simulink model "FullFilterTest_testJ"  (R2020a)
settings: Solver=ode3  StartTime=0.0  StopTime=100  FixedStep=1  RelTol=1e-3
libraries: aerolibconvert2 x1, simulink x1, sharedutil x1, sharedtransform x1
settings Model: Creator=pieterpinson  LastModifiedBy=jamie
settings DataIOCC: SaveFormat=StructureWithTime
settings OptimizationCC: LifeSpan=inf
settings DebuggingCC: SFExecutionAtInitializationDiag=none  ArithmeticOperatorsInVariantConditions=warning
settings HardwareCC: ProdBitPerSizeT=32  ProdBitPerPtrDiffT=32  ProdWordSize=32  ProdHWDeviceType=Specified
settings SFSimCC: CustomCodeUndefinedFunction=UseInterfaceOnly
settings CodeAppCC: StateflowObjectComments=on

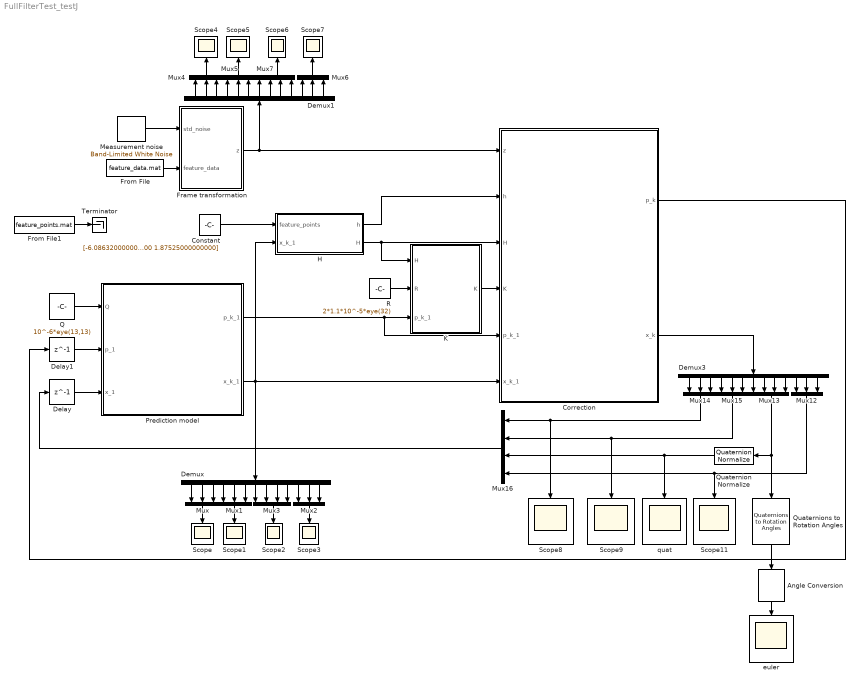
== system FullFilterTest_testJ ==
  Angle Conversion : aerolibconvert2/Angle Conversion  IU=rad  OU=deg
  Constant : Constant  Value=|
      | [-6.08632000000000	-6.29117000000000	-6.23068000000000	-6.17018000000000	0.665410000000000	0.665410000000000	2.50061000000000	2.48017000000000	6.23068000000000	6.35166000000000	6.35166000000000	6.29117000000000	10.8457800000000	10.8280700000000	29.5266400000000	29.5582500000000;
      | -0.635730000000000	1.88967000000000	-0.602200000000000	1.85389000000000	2.17147000000000	2.18343000000000	3.10581000000000	3.09464000000000	-0.636800000000000	2.53604000000000	-0.625630000000000	2.54752000000000	2.60307000000000	1.32946000000000	-8.00742000000000	-9.30518000000000;
      | -1.81476000000000	-1.81476000000000	1.87525000000000	1.93574000000000	7.31953000000000	-7.38003000000000	-7.25904000000000	7.31953000000000	1.93574000000000	2.05673000000000	-1.81476000000000	-1.93574000000000	-3.56903000000000	3.69001000000000	-5.38379000000000	1.87525000000000]
  Correction : MATLAB Function  TreatAsAtomicUnit=on
  Delay : Delay  DelayLength=1  InitialCondition=|
      | [-0.0019 ; 0.0017 ; 1.0891 ; 0 ; 0 ; 0 ; -0.7226 ; 0.6358 ; 0.1434 ; 0.2302
      | ; -0.0873 ; -0.1489 ; 0.0262]
  Delay1 : Delay  DelayLength=1  InitialCondition=100*10*diag([1,1,2,0.01,0.01,0.01,0.01,0.01,0.01,0.01,0.01,0.01,0.01])
  Demux : Demux  Outputs=13
  Demux1 : Demux  Outputs=13
  Demux3 : Demux  Outputs=13
  Frame transformation : MATLAB Function  TreatAsAtomicUnit=on
  From File : FromFile  FileName=feature_data.mat  SampleTime=1
  From File1 : FromFile  FileName=feature_points.mat  SampleTime=0
  H : MATLAB Function  TreatAsAtomicUnit=on
  K : MATLAB Function  TreatAsAtomicUnit=on
  Measurement noise : simulink/Sources/Band-Limited White Noise  Cov=[sin(sin(0.1))]  Ts=1  seed=[23341]
  Mux{,1..2,4..6,12,14..15} (9 alike) : Mux  Inputs=3
  Mux{3,7,13,16} (4 alike) : Mux
  Prediction model : MATLAB Function  TreatAsAtomicUnit=on
  Q : Constant  Value=10^-6*eye(13,13)
  Quaternion Normalize : sharedutil/Quaternion Normalize  aMode=aMode
      settings: SourceProductBaseCode=AE,PW,MT,VE,VP
  Quaternions to Rotation Angles : sharedtransform/Quaternions to Rotation Angles  rotationOrder=ZYX  aMode=aMode
      settings: SourceProductBaseCode=AE,PW,MT,VE,VP
  R : Constant  Value=2*1.1*10^-5*eye(32)
  Scope{,1..9,11} (11 alike) : Scope
  Terminator : Terminator
  euler : Scope
  quat : Scope
  wires:
  Prediction model/2(x_k_1) -> H/2(x_k_1), Correction/6(x_k_1), Demux/1
  Mux3/1 -> Scope2/1
  Demux/13 -> Mux2/3
  Demux/12 -> Mux2/2
  Demux/11 -> Mux2/1
  Demux/10 -> Mux3/4
  Demux/9 -> Mux3/3
  Demux/8 -> Mux3/2
  Demux/7 -> Mux3/1
  Demux/6 -> Mux1/3
  Demux/5 -> Mux1/2
  Demux/4 -> Mux1/1
  Demux/3 -> Mux/3
  Demux/2 -> Mux/2
  Demux/1 -> Mux/1
  Mux1/1 -> Scope1/1
  Mux/1 -> Scope/1
  Delay/1 -> Prediction model/3(x_1)
  Mux2/1 -> Scope3/1
  Q/1 -> Prediction model/1(Q)
  Delay1/1 -> Prediction model/2(p_1)
  Mux6/1 -> Scope7/1
  Demux1/3 -> Mux4/3
  Demux1/10 -> Mux7/4
  Demux1/2 -> Mux4/2
  Demux1/1 -> Mux4/1
  Demux1/11 -> Mux6/1
  Mux4/1 -> Scope4/1
  Mux5/1 -> Scope5/1
  Mux7/1 -> Scope6/1
  Demux1/6 -> Mux5/3
  Demux1/9 -> Mux7/3
  Demux1/13 -> Mux6/3
  Demux1/12 -> Mux6/2
  Demux1/7 -> Mux7/1
  Frame transformation/1(z) -> Correction/1(z), Demux1/1
  Demux1/4 -> Mux5/1
  Demux1/5 -> Mux5/2
  Demux1/8 -> Mux7/2
  H/2(H) -> Correction/3(H), K/1(H)
  Correction/1(p_k) -> Delay1/1
  Correction/2(x_k) -> Demux3/1
  Prediction model/1(p_k_1) -> Correction/5(p_k_1), K/3(p_k_1)
  K/1(K) -> Correction/4(K)
  R/1 -> K/2(R)
  Mux13/1 -> Quaternions to Rotation Angles/1, Quaternion Normalize/1
  Demux3/5 -> Mux15/2
  Demux3/13 -> Mux12/3
  Mux15/1 -> Mux16/2, Scope9/1
  Demux3/9 -> Mux13/3
  Demux3/1 -> Mux14/1
  Demux3/8 -> Mux13/2
  Mux12/1 -> Mux16/4, Scope11/1
  Demux3/6 -> Mux15/3
  Demux3/7 -> Mux13/1
  Demux3/4 -> Mux15/1
  Demux3/2 -> Mux14/2
  Demux3/3 -> Mux14/3
  Demux3/10 -> Mux13/4
  Demux3/12 -> Mux12/2
  Demux3/11 -> Mux12/1
  Quaternion Normalize/1 -> Mux16/3, quat/1
  Mux16/1 -> Delay/1
  Mux14/1 -> Mux16/1, Scope8/1
  H/1(h) -> Correction/2(h)
  Measurement noise/1 -> Frame transformation/1(std_noise)
  From File/1 -> Frame transformation/2(feature_data)
  Constant/1 -> H/1(feature_points)
  From File1/1 -> Terminator/1
  Angle Conversion/1 -> euler/1
  Quaternions to Rotation Angles/1 -> Angle Conversion/1

== matlab function FullFilterTest_testJ/Frame transformation ==
  data: z output; std_noise input; feature_data input
function z = measurements(std_noise,feature_data)
   
    %import and convert featured data points 
    datapoints = feature_data(:,1);
    z = zeros(32,1);
    
    %pixel size
    pixel_size = 1.1*10^-5;
    
    %number of featurepoints
    n = 16;
    
    for i=1:2*n
        datapoints(i) = datapoints(i) + std_noise;
        z(i,1) = pixel_size*(0.5*datapoints(i)+128);
    end
    
end

== matlab function FullFilterTest_testJ/Prediction model ==
  data: Q input; p_1 input; p_k_1 output; x_k_1 output; x_1 input
function [p_k_1,x_k_1]= prediction(Q,p_1,x_1)

%orbital parameter
mu = 3.986*10^14;
R_earth = 6371000;
H_target = 773000;
a = R_earth + H_target;
n = sqrt(mu/(a^3));

%clohessy-wiltshire equations
dr = [4-3*cos(n) 0 0 sin(n)/n 2*(1-cos(n))/n 0 ; 6*(sin(n)-n) 1 0 2*(cos(n)-1)/n (4*sin(n)-3*n)/n 0 ; 0 0 cos(n) 0 0 sin(n)/n];
dv = [3*n*sin(n) 0 0 cos(n) 2*sin(n) 0 ; 6*n*(cos(n)-1) 0 0 -2*sin(n) 4*cos(n)-3 0 ; 0 0 -n*sin(n) 0 0 cos(n)];

%quaternion kinematic equation
dq = 0.5*[0 x_1(13) -x_1(12) x_1(11) ; -x_1(13) 0 x_1(11) x_1(12) ; x_1(12) -x_1(11) 0 x_1(13) ; -x_1(11) -x_1(12) -x_1(13) 0];

%state transition matrix
fi = [dr zeros(3,7) ; dv zeros(3,7) ; zeros(4,6) dq zeros(4,3) ; zeros(3,10) eye(3)];

%propogation step
x_k_1 = [0;0;0;0;0;0;x_1(7:10);0;0;0] + fi * x_1;
p_k_1 = fi * p_1 * fi.' + Q;

end


%dq1 = 0.5*[x_1(10) -x_1(9) x_1(8) x_1(7) ; x_1(9) x_1(10) -x_1(7) x_1(8) ; -x_1(8) x_1(7) x_1(10) x_1(9) ; -x_1(7) -x_1(8) -x_1(9) x_1(10)];
%fi(7,7) = x_1(7) + 0.5*(x_1(12)*x_1(8) - x_1(12)*x_1(9) + x_1(11)*x_1(10));
%fi(8,8) = x_1(8) + 0.5*(-x_1(13)*x_1(7) + x_1(11)*x_1(9) + x_1(12)*x_1(10));
%fi(9,9) = x_1(9) + 0.5*(x_1(12)*x_1(7) - x_1(11)*x_1(8) + x_1(13)*x_1(10));
%fi(10,10) = x_1(10) + 0.5*(-x_1(11)*x_1(7) - x_1(12)*x_1(8) - x_1(13)*x_1(9));

== matlab function FullFilterTest_testJ/Correction ==
  data: z input; h input; p_k output; x_k output; H input; K input; p_k_1 input; x_k_1 input
function [p_k,x_k]= correction(z,h,H,K,p_k_1,x_k_1)

%correction step
x_k = x_k_1 + K*(z - h);
p_k = (eye(13,13) - K*H)*p_k_1;

end

== matlab function FullFilterTest_testJ/H ==
  data: feature_points input; h output; x_k_1 input; H output
function [h,H]= Jacobian(feature_points,x_k_1)
    
    %focal length of the camera
    fx = 3.9*10^-3;
    fy = 3.9*10^-3;
    
    %pixelsize
    pixel_size = 1.1*10^-5;
    
    %number of featurepoints
    n = 16;

    %individual vector definition
    vectorJacobian = zeros(2*n, 3);
    quaternionJacobian = zeros(2*n, 4);
    h = zeros(32,1);
    
    %import and convert featured data points
    wireframe = feature_points;
    
    for i = 1:n
        
        %quaternion rotation matrix
        q = x_k_1(7:10);
        R_q = [q(1)^2+q(2)^2-q(3)^2-q(3)^2 2*(q(2)*q(3)-q(1)*q(4)) 2*(q(4)*q(2)+q(1)*q(3));
         2*(q(2)*q(3)+q(1)*q(4)) q(1)^2-q(2)^2+q(3)^2-q(4)^2 2*(q(3)*q(4)-q(1)*q(2));
         2*(q(4)*q(2)-q(1)*q(3)) 2*(q(3)*q(4)+q(1)*q(2)) q(1)^2-q(2)^2-q(3)^2+q(4)^2];
        
        %position vector
        xyz = R_q*wireframe(:,i)+x_k_1(1:3);
        
        %h vector calculation
        h(2*i-1,1) = xyz(1)/xyz(3)*fx+256*pixel_size;
        h(2*i,1) = xyz(2)/xyz(3)*fy+256*pixel_size;
        
        %position Jacobian calculation
        vectorJacobian(i*2-1:i*2,1:3) = [fx/xyz(3) 0 -fx*xyz(1)/xyz(3)^2 ; 0 fy/xyz(3) -fy*xyz(2)/xyz(3)^2];
        
        %quaternion rotation Jacobian calculation
        dH_dq_1 = [2*q(1) -2*q(4) 2*q(3); 2*q(4) 2*q(1) -2*q(2); -2*q(3) 2*q(2) 2*q(1)]*xyz;
        dH_dq_2 = [2*q(2) 2*q(3) 2*q(4); 2*q(3) -2*q(2) -2*q(1); 2*q(4) 2*q(1) -2*q(2)]*xyz;
        dH_dq_3 = [-2*q(3) 2*q(2) 2*q(1); 2*q(2) 2*q(3) 2*q(4); -2*q(1) 2*q(4) -2*q(3)]*xyz;
        dH_dq_4 = [-2*q(4) -2*q(1) 2*q(2); 2*q(1) -2*q(4) 2*q(3); 2*q(1) 2*q(3) 2*q(4)]*xyz;
        dH_dq = [dH_dq_1 dH_dq_2 dH_dq_3 dH_dq_4] * [1 0 0 0; 0 -1 0 0; 0 0 -1 0; 0 0 0 -1];
        
        quaternionJacobian(i*2-1:i*2,1:4) = vectorJacobian(i*2-1:i*2,1:3)*dH_dq;
        
    end
    
    %final Jacobian vector
    H = [vectorJacobian, zeros(2*n, 3), quaternionJacobian, zeros(2*n, 3)];

end

== matlab function FullFilterTest_testJ/K ==
  data: H input; R input; K output; p_k_1 input
function K = kalmangain(H,R,p_k_1)

%kalman gain calculation
K = p_k_1 * H' * inv(H * p_k_1 * H' + R);

end
